simulink model "SOC_Calc202510082250"  (R2025a)
settings: Solver=VariableStepAuto  StartTime=0.0  StopTime=100  RelTol=1e-3
undefined symbols (not defined in the file): DiscIntNeverNeededParam
settings Model: Creator=86138  LastModifiedBy=86138
settings DataIOCC: ReturnWorkspaceOutputs=off

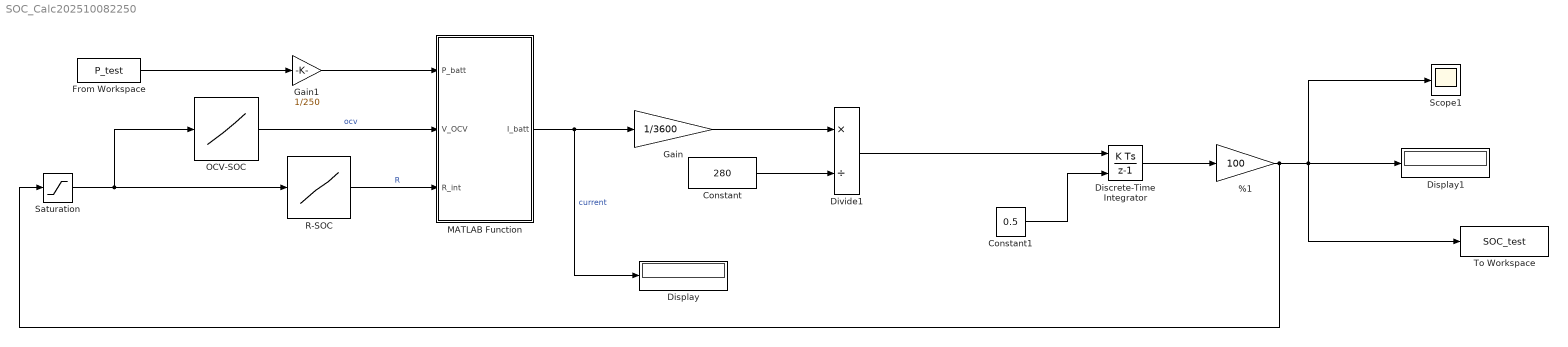
== system SOC_Calc202510082250 ==
  %1 : Gain  Gain=100
  Constant : Constant  Value=280
  Constant1 : Constant  Value=0.5
  Discrete-Time Integrator : DiscreteIntegrator  InitialConditionSource=external  SampleTime=-1  ICPrevOutput=DiscIntNeverNeededParam  ICPrevScaledInput=DiscIntNeverNeededParam
  Display : Display
  Display1 : Display
  Divide1 : Product  Inputs=*/
  From Workspace : FromWorkspace  VariableName=P_test
  Gain : Gain  Gain=1/3600
  Gain1 : Gain  Gain=1/250
  MATLAB Function : MATLAB Function  TreatAsAtomicUnit=on
  OCV-SOC : Lookup_n-D  NumberOfTableDimensions=1  BreakpointsForDimension1=[-5:5]  Table=tanh([-5:5])  InternalRulePriority=Speed  RndMeth=Simplest
  R-SOC : Lookup_n-D  NumberOfTableDimensions=1  BreakpointsForDimension1=[-5:5]  Table=tanh([-5:5])  InternalRulePriority=Speed  RndMeth=Simplest
  Saturation : Saturate  UpperLimit=100  LowerLimit=0
  Scope1 : Scope
      settings: ActiveDisplayYMinimum=-125.99987011909816  ActiveDisplayYMaximum=215.17892908104051
  To Workspace : ToWorkspace  VariableName=SOC_test  SaveFormat=Timeseries  SampleTime=-1
  wires:
  OCV-SOC/1 -> MATLAB Function/2(V_OCV)  "ocv"
  Discrete-Time Integrator/1 -> %1/1
  Gain/1 -> Divide1/1
  R-SOC/1 -> MATLAB Function/3(R_int)  "R"
  Constant/1 -> Divide1/2
  Divide1/1 -> Discrete-Time Integrator/1
  Saturation/1 -> R-SOC/1, OCV-SOC/1
  Constant1/1 -> Discrete-Time Integrator/2
  %1/1 -> Saturation/1, Scope1/1, Display1/1, To Workspace/1
  From Workspace/1 -> Gain1/1
  Gain1/1 -> MATLAB Function/1(P_batt)
  MATLAB Function/1(I_batt) -> Gain/1, Display/1  "current"

== matlab function SOC_Calc202510082250/MATLAB Function ==
  data: P_batt input; V_OCV input; R_int input; I_batt output
function I_batt = fcn(P_batt, V_OCV, R_int)
% =========================================================================
% 功能: 根据单电芯功率、开路电压和内阻计算电池电流
% 模型: V_term = V_OCV + I_batt * R_int (一阶ECM)
% 约定: 电流 I_batt > 0 表示充电, I_batt < 0 表示放电
% -------------------------------------------------------------------------
% 输入:
%   P_batt: 单个电芯的功率 (W)。P_batt > 0 表示充电, P_batt < 0 表示放电。
%           (注意: 这是从系统总功率缩放后的值)
%   V_OCV:  当前SOC下的单电芯开路电压 (V)。
%   R_int:  当前SOC和SOH下的单电芯等效内阻 (Ohm)。
% -------------------------------------------------------------------------
% 输出:
%   I_batt: 计算出的单电芯电流 (A)。
% =========================================================================

    % 物理方程推导:
    % 1) P_batt = V_term * I_batt
    % 2) V_term = V_OCV + I_batt * R_int  =>  I_batt = (V_term - V_OCV) / R_int
    % 将 (2) 代入 (1):
    % P_batt = V_term * (V_term - V_OCV) / R_int
    % 整理得到关于 V_term 的一元二次方程:
    % V_term^2 - V_OCV * V_term - P_batt * R_int = 0

    % -- 步骤 1: 计算一元二次方程的判别式 --
    % 判别式 delta = b^2 - 4ac, 其中 a=1, b=-V_OCV, c=-P_batt*R_int
    discriminant = V_OCV^2 + 4 * P_batt * R_int;

    % -- 步骤 2: 检查解的物理可行性 --
    % 如果判别式小于0，意味着在当前 V_OCV 和 R_int 条件下，电池无法
    % 提供或吸收这么大的功率，方程没有实数解。这通常发生在请求的
    % 放电功率超过了电池的最大输出功率 P_max = V_OCV^2 / (4*R_int)。
    % 在这种情况下，我们将电流视为0，模拟BMS的功率限制行为。
    if discriminant < 0
        I_batt = 0; % 功率请求超出物理极限，返回0电流
        % 在实际应用中，此处可以增加一个警告标志输出
        return; % 提前退出函数
    end

    % -- 步骤 3: 求解端电压 V_term --
    % 根据求根公式 V_term = (-b ± sqrt(delta)) / 2a
    % V_term = (V_OCV ± sqrt(discriminant)) / 2
    % 我们需要选择物理上有意义的解。
    % 充电时 (P_batt > 0), V_term > V_OCV。
    % 放电时 (P_batt < 0), V_term < V_OCV。
    % 经过分析，使用 "+" 号的解在两种情况下都能满足物理约束。
    V_term = (V_OCV + sqrt(discriminant)) / 2;

    % -- 步骤 4: 计算电流 I_batt --
    % 为避免当 R_int 极小时可能出现的数值不稳定问题，我们进行一个简单的检查。
    if R_int < 1e-6 % 避免除以一个非常小的数或零
        % 如果内阻几乎为0, 则 V_term 约等于 V_OCV。
        if abs(V_OCV) > 1e-6
            I_batt = P_batt / V_OCV;
        else
            I_batt = 0; % V_OCV也为0，无法计算
        end
    else
        % 使用 V_term = V_OCV + I_batt * R_int 的变形公式计算电流。
        % 这比 I_batt = P_batt / V_term 在数值上更稳定。
        I_batt = (V_term - V_OCV) / R_int;
    end
end
